simulink model "Simulacao"  (R2014a)
settings: Solver=ode45  StartTime=0.0  StopTime=200  RelTol=1e-3
libraries: dspsrcs4 x1, simulink x1
settings Model: Creator=Sillas  LastModifiedBy=Sillas

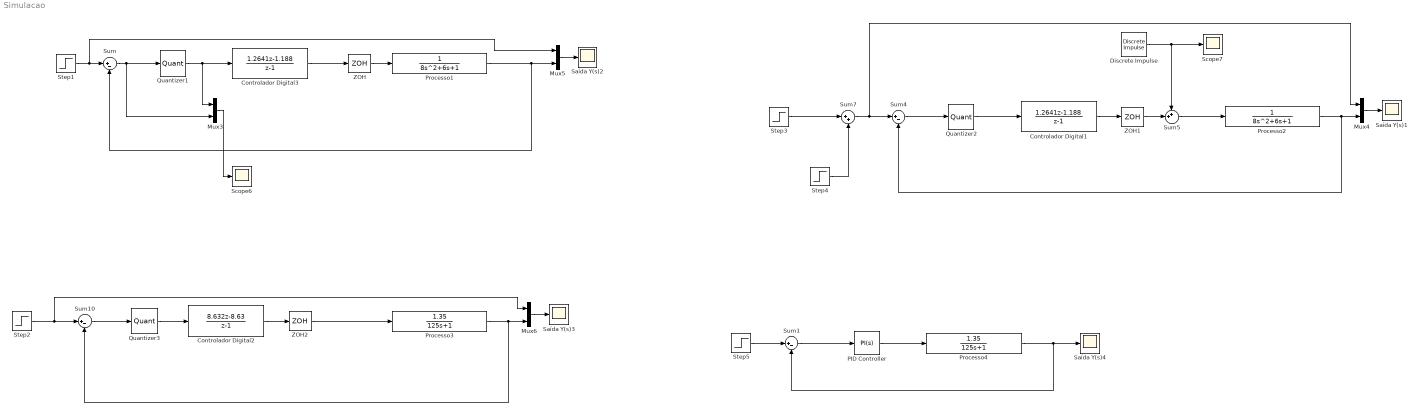
== system Simulacao ==
  Controlador Digital1 : DiscreteTransferFcn  Numerator=[1.2641 -1.188]  Denominator=[1 -1]  SampleTime=0.3
  Controlador Digital2 : DiscreteTransferFcn  Numerator=[8.632 -8.63]  Denominator=[1 -1]  SampleTime=0.01
  Controlador Digital3 : DiscreteTransferFcn  Numerator=[1.2641 -1.188]  Denominator=[1 -1]  SampleTime=0.3
  Discrete Impulse : dspsrcs4/Discrete  Impulse  Delay=3  SampleTime=0.3  FrameSample=1  dataType=double  isSigned=on  wordLen=16  udDataType=sfix(16)  fracBitsMode=Best precision  numFracBits=15  OutDataTypeStr=double  LastOutDataTypeStr=double
  Mux{3..6} (4 alike) : Mux  Inputs=2
  PID Controller : simulink/Continuous/PID Controller  Controller=PI  TimeDomain=Continuous-time  SampleTime=1  IntegratorMethod=Forward Euler  FilterMethod=Forward Euler  Form=Parallel  P=6.01638469278482  I=0.0550885441561822  D=0  N=100  InitialConditionSource=internal  InitialConditionForIntegrator=0  InitialConditionForFilter=0  ExternalReset=none  LimitOutput=off  UpperSaturationLimit=inf  LowerSaturationLimit=-inf  LinearizeAsGain=on  AntiWindupMode=none  Kb=1  TrackingMode=off  Kt=1  PParamMin=[]  PParamMax=[]  IParamMin=[]  IParamMax=[]  DParamMin=[]  DParamMax=[]  NParamMin=[]  NParamMax=[]  KbParamMin=[]  KbParamMax=[]  KtParamMin=[]  KtParamMax=[]  POutMin=[]  POutMax=[]  IOutMin=[]  IOutMax=[]  DOutMin=[]  DOutMax=[]  NOutMin=[]  NOutMax=[]  KbOutMin=[]  KbOutMax=[]  KtOutMin=[]  KtOutMax=[]  IntegratorOutMin=[]  IntegratorOutMax=[]  FilterOutMin=[]  FilterOutMax=[]  SumOutMin=[]  SumOutMax=[]  SumI1OutMin=[]  SumI1OutMax=[]  SumI2OutMin=[]  SumI2OutMax=[]  SumI3OutMin=[]  SumI3OutMax=[]  SumDOutMin=[]  SumDOutMax=[]  SaturationOutMin=[]  SaturationOutMax=[]  IntegratorContinuousStateAttributes=''  IntegratorStateMustResolveToSignalObject=off  IntegratorRTWStateStorageClass=Auto  FilterContinuousStateAttributes=''  FilterStateMustResolveToSignalObject=off  FilterRTWStateStorageClass=Auto
  Processo1 : TransferFcn  Denominator=[8 6 1]
  Processo2 : TransferFcn  Denominator=[8 6 1]
  Processo3 : TransferFcn  Numerator=[1.35]  Denominator=[125 1]
  Processo4 : TransferFcn  Numerator=[1.35]  Denominator=[125 1]
  Quantizer1 : Quantizer  QuantizationInterval=0.1  LinearizeAsGain=off  SampleTime=0.3
  Quantizer2 : Quantizer  QuantizationInterval=0.3  LinearizeAsGain=off  SampleTime=0.3
  Quantizer3 : Quantizer  QuantizationInterval=0.001  LinearizeAsGain=off  SampleTime=0.01
  Saída Y(s){1..4} (4 alike) : Scope
      Saída Y(s)1 settings: SaveName=grafico1
      Saída Y(s)2 settings: SaveName=grafico
      Saída Y(s)3 settings: SaveName=grafico2
      Saída Y(s)4 settings: SaveName=grafico3
  Scope6 : Scope
      settings: SaveName=ScopeData7
  Scope7 : Scope
  Step{1..3,5} (4 alike) : Step  Time=0  SampleTime=0
  Step4 : Step  Time=12  SampleTime=0
  Sum{,1,4,10} (4 alike) : Sum  Inputs=|+-
  Sum5 : Sum  Inputs=++|
  Sum7 : Sum  Inputs=|++
  ZOH : ZeroOrderHold  SampleTime=0.3
  ZOH1 : ZeroOrderHold  SampleTime=0.3
  ZOH2 : ZeroOrderHold  SampleTime=0.01
  wires:
  Step1/1 -> Mux5/1, Sum/1
  ZOH/1 -> Processo1/1
  Sum/1 -> Mux3/2, Quantizer1/1
  Mux3/1 -> Scope6/1
  Quantizer1/1 -> Controlador Digital3/1, Mux3/1
  Controlador Digital3/1 -> ZOH/1
  Sum4/1 -> Quantizer2/1
  Quantizer2/1 -> Controlador Digital1/1
  Controlador Digital1/1 -> ZOH1/1
  Processo2/1 -> Sum4/2, Mux4/2
  Mux4/1 -> Saída Y(s)1/1
  Processo1/1 -> Sum/2, Mux5/2
  Mux5/1 -> Saída Y(s)2/1
  Discrete Impulse/1 -> Sum5/1, Scope7/1
  ZOH1/1 -> Sum5/2
  Sum5/1 -> Processo2/1
  Step3/1 -> Sum7/1
  Step4/1 -> Sum7/2
  Sum7/1 -> Mux4/1, Sum4/1
  Sum10/1 -> Quantizer3/1
  Quantizer3/1 -> Controlador Digital2/1
  Controlador Digital2/1 -> ZOH2/1
  Processo3/1 -> Sum10/2, Mux6/2
  Mux6/1 -> Saída Y(s)3/1
  ZOH2/1 -> Processo3/1
  Step2/1 -> Mux6/1, Sum10/1
  Step5/1 -> Sum1/1
  Processo4/1 -> Sum1/2, Saída Y(s)4/1
  Sum1/1 -> PID Controller/1
  PID Controller/1 -> Processo4/1
